simulink model "HighPassFilter"  (R2020b)
settings: Solver=VariableStepAuto  StartTime=0.0  StopTime=0.01  RelTol=1e-3
settings Model: Creator=vigne  LastModifiedBy=prabhudevmaddipudi

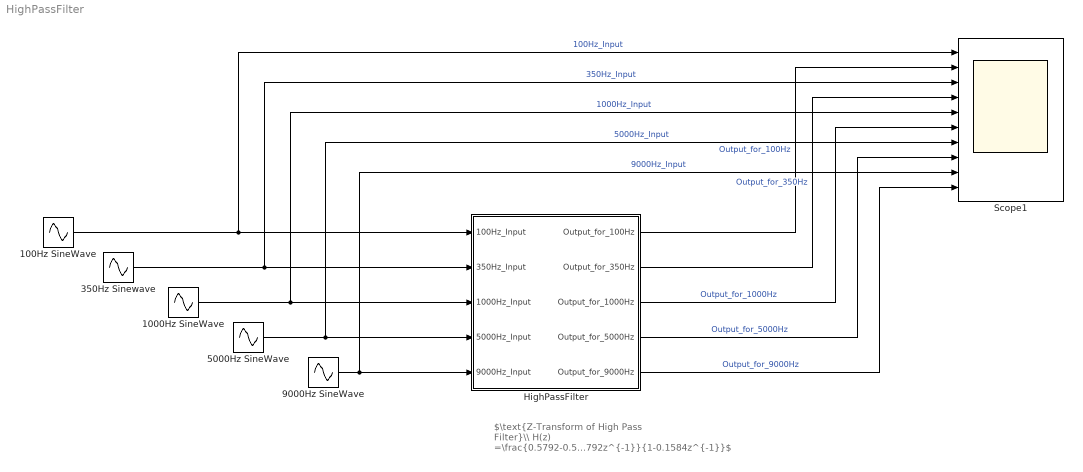
== system HighPassFilter ==
  note: $\text{Z-Transform of High Pass Filter}\\ H(z) =\frac{0.5792-0.5792z^{-1}}{1-0.1584z^{-1}}$
  1000Hz SineWave : Sin  Frequency=2*pi*1000  SampleTime=0
  100Hz SineWave : Sin  Frequency=2*pi*100  SampleTime=0
  350Hz Sinewave : Sin  Frequency=2*pi*350  SampleTime=0
  5000Hz SineWave : Sin  Frequency=2*pi*5000  SampleTime=0
  9000Hz SineWave : Sin  Frequency=2*pi*9000  SampleTime=0
  HighPassFilter : Subsystem
  Scope1 : Scope  NumInputPorts=10
  wires:
  100Hz SineWave/1 -> Scope1/1, HighPassFilter/1(100Hz_Input)  "100Hz_Input"
  350Hz Sinewave/1 -> Scope1/3, HighPassFilter/2(350Hz_Input)  "350Hz_Input"
  1000Hz SineWave/1 -> Scope1/5, HighPassFilter/3(1000Hz_Input)  "1000Hz_Input"
  5000Hz SineWave/1 -> Scope1/7, HighPassFilter/4(5000Hz_Input)  "5000Hz_Input"
  9000Hz SineWave/1 -> Scope1/9, HighPassFilter/5(9000Hz_Input)  "9000Hz_Input"
  HighPassFilter/1(Output_for_100Hz) -> Scope1/2  "Output_for_100Hz"
  HighPassFilter/2(Output_for_350Hz) -> Scope1/4  "Output_for_350Hz"
  HighPassFilter/3(Output_for_1000Hz) -> Scope1/6  "Output_for_1000Hz"
  HighPassFilter/4(Output_for_5000Hz) -> Scope1/8  "Output_for_5000Hz"
  HighPassFilter/5(Output_for_9000Hz) -> Scope1/10  "Output_for_9000Hz"

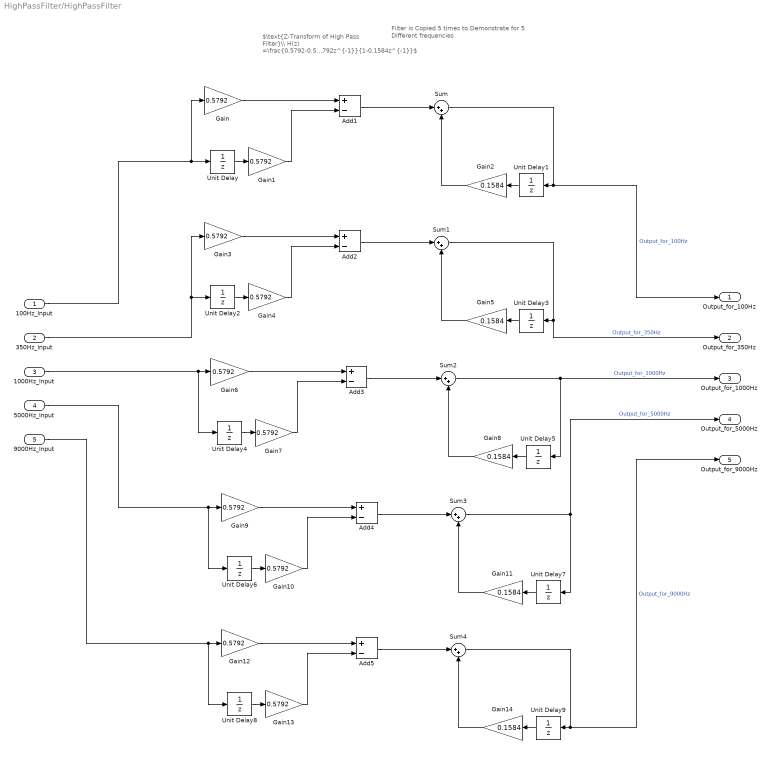
== system HighPassFilter/HighPassFilter ==
  note: Filter is Copied 5 times to Demonstrate for
      | 5 Different frequencies
  note: $\text{Z-Transform of High Pass Filter}\\ H(z) =\frac{0.5792-0.5792z^{-1}}{1-0.1584z^{-1}}$
  100Hz_Input : Inport
  350Hz_Input : Inport  Port=2
  1000Hz_Input : Inport  Port=3
  5000Hz_Input : Inport  Port=4
  9000Hz_Input : Inport  Port=5
  Add{1..5} (5 alike) : Sum  Inputs=+-
  Gain{,1,3..4,6..7,9..10,12..13} (10 alike) : Gain  Gain=0.5792
  Gain{2,5,8,11,14} (5 alike) : Gain  Gain=0.1584
  Sum{,1..4} (5 alike) : Sum  Inputs=|++
  Unit Delay{,1..9} (10 alike) : UnitDelay  SampleTime=-1  HasFrameUpgradeWarning=on
  Output_for_100Hz : Outport
  Output_for_350Hz : Outport  Port=2
  Output_for_1000Hz : Outport  Port=3
  Output_for_5000Hz : Outport  Port=4
  Output_for_9000Hz : Outport  Port=5
  wires:
  1000Hz_Input/1 -> Unit Delay4/1, Gain6/1
  Unit Delay2/1 -> Gain4/1
  Gain/1 -> Add1/1
  Unit Delay/1 -> Gain1/1
  Gain2/1 -> Sum/2
  Sum/1 -> Output_for_100Hz/1, Unit Delay1/1  "Output_for_100Hz"
  Gain9/1 -> Add4/1
  9000Hz_Input/1 -> Unit Delay8/1, Gain12/1
  Sum4/1 -> Unit Delay9/1, Output_for_9000Hz/1  "Output_for_9000Hz"
  Unit Delay7/1 -> Gain11/1
  5000Hz_Input/1 -> Unit Delay6/1, Gain9/1
  Add3/1 -> Sum2/1
  Sum1/1 -> Unit Delay3/1, Output_for_350Hz/1  "Output_for_350Hz"
  350Hz_Input/1 -> Gain3/1, Unit Delay2/1
  Unit Delay8/1 -> Gain13/1
  Add2/1 -> Sum1/1
  Gain1/1 -> Add1/2
  Unit Delay1/1 -> Gain2/1
  Sum3/1 -> Unit Delay7/1, Output_for_5000Hz/1  "Output_for_5000Hz"
  Add4/1 -> Sum3/1
  Unit Delay3/1 -> Gain5/1
  Gain6/1 -> Add3/1
  Gain4/1 -> Add2/2
  Gain3/1 -> Add2/1
  Unit Delay4/1 -> Gain7/1
  100Hz_Input/1 -> Gain/1, Unit Delay/1
  Gain7/1 -> Add3/2
  Unit Delay5/1 -> Gain8/1
  Gain13/1 -> Add5/2
  Gain12/1 -> Add5/1
  Add5/1 -> Sum4/1
  Sum2/1 -> Unit Delay5/1, Output_for_1000Hz/1  "Output_for_1000Hz"
  Gain14/1 -> Sum4/2
  Gain5/1 -> Sum1/2
  Gain10/1 -> Add4/2
  Unit Delay9/1 -> Gain14/1
  Gain8/1 -> Sum2/2
  Gain11/1 -> Sum3/2
  Unit Delay6/1 -> Gain10/1
  Add1/1 -> Sum/1
